simulink model "reduce_obse"  (R2020a)
settings: Solver=VariableStepAuto  StartTime=0.0  StopTime=10.0  RelTol=1e-3
values from neighbouring files (symbols this model uses):
  K1 = real(K1)    [observa.m]
undefined symbols (not defined in the file or in its folder): A, B, C, D1, E, G, H, x0
settings Model: Creator=wyton  LastModifiedBy=wyton

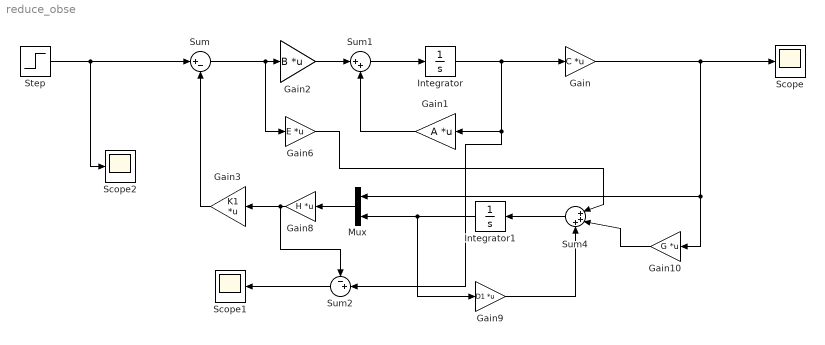
== system reduce_obse ==
  Gain : Gain  Gain=C  Multiplication=Matrix(K*u)
      settings: AttributesFormatString=C
  Gain1 : Gain  Gain=A  Multiplication=Matrix(K*u)
      settings: AttributesFormatString=A
  Gain10 : Gain  Gain=G  Multiplication=Matrix(K*u)
  Gain2 : Gain  Tag=B  Gain=B  Multiplication=Matrix(K*u)
      settings: AttributesFormatString=B
  Gain3 : Gain  Gain=K1  Multiplication=Matrix(K*u)
      settings: AttributesFormatString=K
  Gain6 : Gain  Gain=E  Multiplication=Matrix(K*u)
  Gain8 : Gain  Gain=H  Multiplication=Matrix(K*u)
  Gain9 : Gain  Gain=D1  Multiplication=Matrix(K*u)
  Integrator : Integrator  InitialCondition=x0
  Integrator1 : Integrator
  Mux : Mux  Inputs=2
  Scope : Scope
      settings: AttributesFormatString=output
  Scope1 : Scope
      settings: AttributesFormatString=state error
  Scope2 : Scope
  Step : Step  Time=0  After=0  SampleTime=0
  Sum : Sum  Inputs=|+-
  Sum1 : Sum  Inputs=|++
  Sum2 : Sum  Inputs=-+|
  Sum4 : Sum  Inputs=|+++
  wires:
  Step/1 -> Scope2/1, Sum/1
  Sum/1 -> Gain6/1, Gain2/1
  Sum1/1 -> Integrator/1
  Gain2/1 -> Sum1/1
  Integrator/1 -> Sum2/2, Gain1/1, Gain/1
  Gain1/1 -> Sum1/2
  Gain/1 -> Gain10/1, Mux/1, Scope/1
  Gain3/1 -> Sum/2
  Gain8/1 -> Sum2/1, Gain3/1
  Mux/1 -> Gain8/1
  Integrator1/1 -> Gain9/1, Mux/2
  Sum4/1 -> Integrator1/1
  Gain9/1 -> Sum4/3
  Gain10/1 -> Sum4/2
  Gain6/1 -> Sum4/1
  Sum2/1 -> Scope1/1
